simulink model "for_using_function"  (R2021a)
settings: Solver=VariableStepAuto  StartTime=0.0  StopTime=10.0  RelTol=1e-3
settings Model: Creator=Acer  LastModifiedBy=Acer

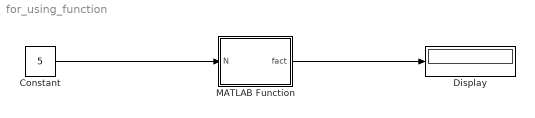
== system for_using_function ==
  Constant : Constant  Value=5
  Display : Display
  MATLAB Function : MATLAB Function  TreatAsAtomicUnit=on
  wires:
  Constant/1 -> MATLAB Function/1(N)
  MATLAB Function/1(fact) -> Display/1

== matlab function for_using_function/MATLAB Function ==
  data: N input; fact output
function fact = fcn(N)
fact=1;
for i=1:N
    fact=fact*i;
end
end
